simulink model "lab2_2"  (R2020b)
settings: Solver=VariableStepAuto  StartTime=0.0  StopTime=30  MaxStep=0.01  RelTol=1e-3
InitFcn:
  | lambda = 5;
  | theta = 5;
settings Model: Creator=Eeer12  LastModifiedBy=Eugene

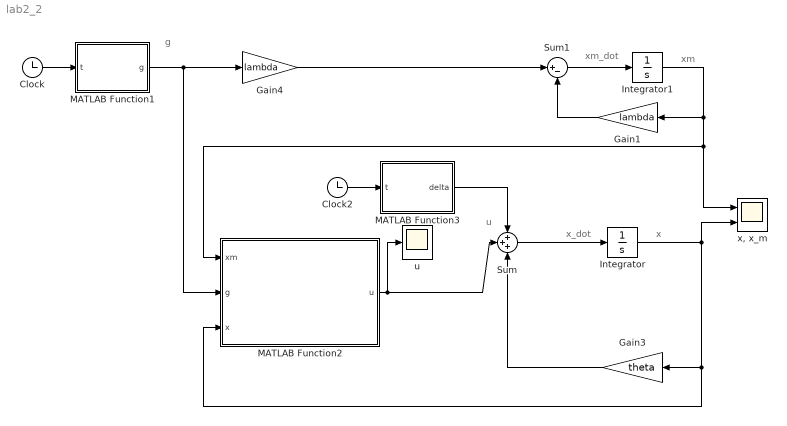
== system lab2_2 ==
  note: g
  note: u
  note: x_dot
  note: x
  note: xm_dot
  note: xm
  Clock : Clock
  Clock2 : Clock
  Gain1 : Gain  Gain=lambda
  Gain3 : Gain  Gain=theta
  Gain4 : Gain  Gain=lambda
  Integrator : Integrator  InitialCondition=1
  Integrator1 : Integrator
  MATLAB Function1 : MATLAB Function  TreatAsAtomicUnit=on
  MATLAB Function2 : MATLAB Function  TreatAsAtomicUnit=on
  MATLAB Function3 : MATLAB Function  TreatAsAtomicUnit=on
  Sum : Sum  Inputs=+++
  Sum1 : Sum  Inputs=|+-
  u : Scope
  "x, x_m" : Scope  NumInputPorts=2
  wires:
  Integrator/1 -> "x, x_m"/2, MATLAB Function2/3(x), Gain3/1
  Sum/1 -> Integrator/1
  Gain1/1 -> Sum1/2
  Sum1/1 -> Integrator1/1
  Clock/1 -> MATLAB Function1/1(t)
  Integrator1/1 -> "x, x_m"/1, MATLAB Function2/1(xm), Gain1/1
  Gain4/1 -> Sum1/1
  Clock2/1 -> MATLAB Function3/1(t)
  Gain3/1 -> Sum/3
  MATLAB Function2/1(u) -> Sum/2, u/1
  MATLAB Function3/1(delta) -> Sum/1
  MATLAB Function1/1(g) -> MATLAB Function2/2(g), Gain4/1

== matlab function lab2_2/MATLAB Function1 ==
  data: t input; g output
function g = fcn(t)

g = 2*sin(5*t);

== matlab function lab2_2/MATLAB Function2 ==
  data: xm input; g input; x input; u output; lambda parameter
function u  = fcn(xm, g, x, lambda)

gamma = 100;
e = xm - x;
theta_hat = -gamma*x*e;
u = -theta_hat*x - lambda*x + lambda*g;

== matlab function lab2_2/MATLAB Function3 ==
  data: t input; delta output; theta parameter
function delta = fcn(t, theta)

delta = (1 + t)^(-1/8) * (1 - theta*(1 + t)^(-1/4) - 3/8*(1 + t)^(-5/4));
